simulink model "singleIntegratorControl"  (R2015b)
settings: Solver=ode8  StartTime=0.0  StopTime=10  FixedStep=0.01  RelTol=1e-3
settings Model: Creator=E183308  LastModifiedBy=E183308

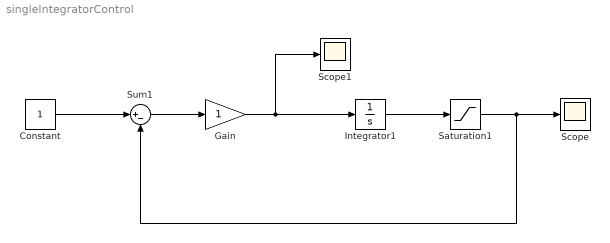
== system singleIntegratorControl ==
  Constant : Constant
  Gain : Gain
  Integrator1 : Integrator
  Saturation1 : Saturate  UpperLimit=0.9  LowerLimit=-0.9
  Scope : Scope
  Scope1 : Scope
  Sum1 : Sum  Inputs=|+-
  wires:
  Integrator1/1 -> Saturation1/1
  Constant/1 -> Sum1/1
  Sum1/1 -> Gain/1
  Gain/1 -> Integrator1/1, Scope1/1
  Saturation1/1 -> Scope/1, Sum1/2
